simulink model "CATSS_Functional"  (R2025b)
settings: Solver=VariableStepAuto  StartTime=0.0  StopTime=10.0  RelTol=1e-3
settings Model: DataDictionary=CATSS_FunctionalInterfaces.sldd  Creator=sarah  LastModifiedBy=sarah

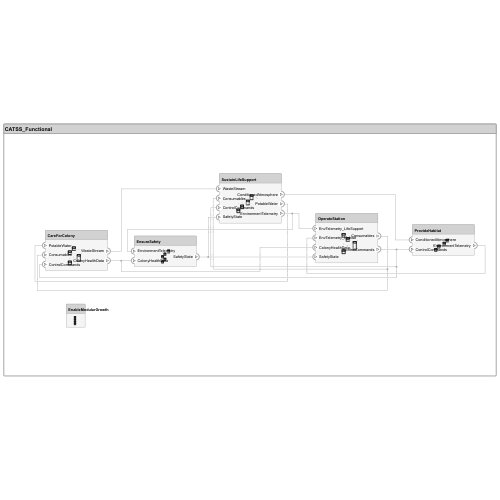
[thumbnail: Simulink's stored preview of the top-level diagram]
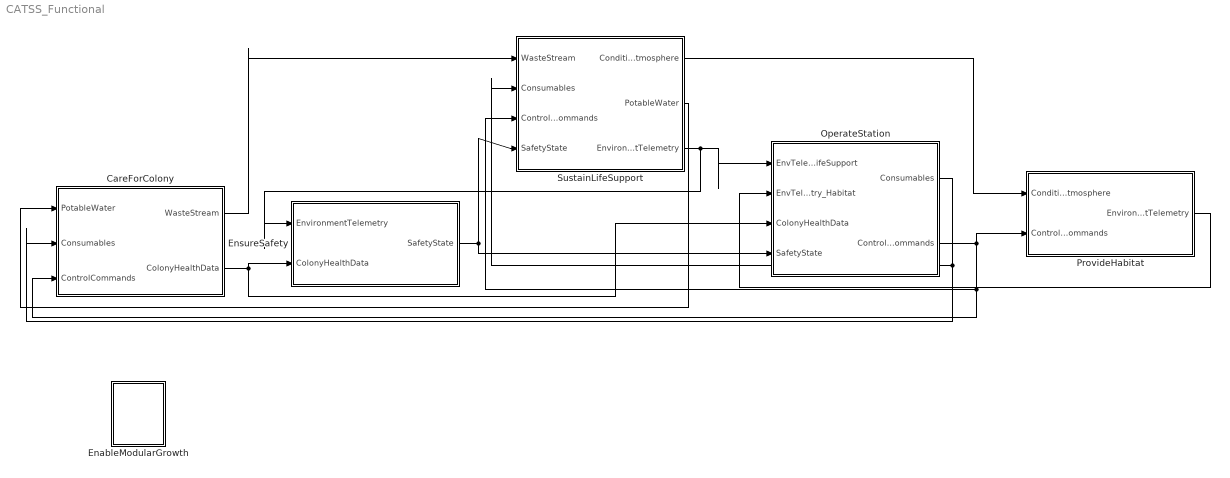
== system CATSS_Functional ==
  CareForColony : Subsystem
      settings: PortSchema="{\"entries\":[{\"content\":{\"headerSize\":26,\"margin\":15,\"minimumSpacing\":25,\"sides\":[{\"content\":{\"connectorIds\":[\"In1\",\"In2\",\"In3\"]},\"type\":\"ConnectorPlacement.EquallySpacedRectSide\",\"uuid\":\"ee9d823c-b058-498d-a1d2-354a2dfab86e\"},{\"content\":{\"connectorIds\":[\"Out1\",\"Out2\"],\"side\":\"RIGHT\"},\"type\":\"ConnectorPlacement.EquallySpacedRectSide\",\"uuid\":\"e3604748-6574-46d6-a392-50dc4429d0e1\"},{\"content\":{\"side\":\"TOP\"},\"type\":\"ConnectorPlacement.EquallySpacedRectSide\",\"uuid\":\"eee796a1-5b1d-4047-be0b-af9e6bf06bf5\"}]},\"type\":\"ConnectorPlacement.EquallySpacedConnector\",\"uuid\":\"95a9b6eb-cbb6-45d0-9b2f-8eab5ca43efc\"}],\"packageUris\":[\"http://schema.mathworks.com/mf0/Connector/R2020b\"],\"version\":\"1.0\"}"
  EnableModularGrowth : Subsystem
      settings: PortSchema="{\"entries\":[{\"content\":{\"headerSize\":26,\"margin\":15,\"minimumSpacing\":25,\"sides\":[{\"content\":{},\"type\":\"ConnectorPlacement.EquallySpacedRectSide\",\"uuid\":\"ee9d823c-b058-498d-a1d2-354a2dfab86e\"},{\"content\":{\"side\":\"RIGHT\"},\"type\":\"ConnectorPlacement.EquallySpacedRectSide\",\"uuid\":\"e3604748-6574-46d6-a392-50dc4429d0e1\"},{\"content\":{\"side\":\"TOP\"},\"type\":\"ConnectorPlacement.EquallySpacedRectSide\",\"uuid\":\"eee796a1-5b1d-4047-be0b-af9e6bf06bf5\"}]},\"type\":\"ConnectorPlacement.EquallySpacedConnector\",\"uuid\":\"95a9b6eb-cbb6-45d0-9b2f-8eab5ca43efc\"}],\"packageUris\":[\"http://schema.mathworks.com/mf0/Connector/R2020b\"],\"version\":\"1.0\"}"
  EnsureSafety : Subsystem
      settings: PortSchema="{\"entries\":[{\"content\":{\"headerSize\":26,\"margin\":15,\"minimumSpacing\":25,\"sides\":[{\"content\":{\"connectorIds\":[\"In1\",\"In2\"]},\"type\":\"ConnectorPlacement.EquallySpacedRectSide\",\"uuid\":\"ee9d823c-b058-498d-a1d2-354a2dfab86e\"},{\"content\":{\"connectorIds\":[\"Out1\"],\"side\":\"RIGHT\"},\"type\":\"ConnectorPlacement.EquallySpacedRectSide\",\"uuid\":\"e3604748-6574-46d6-a392-50dc4429d0e1\"},{\"content\":{\"side\":\"TOP\"},\"type\":\"ConnectorPlacement.EquallySpacedRectSide\",\"uuid\":\"eee796a1-5b1d-4047-be0b-af9e6bf06bf5\"}]},\"type\":\"ConnectorPlacement.EquallySpacedConnector\",\"uuid\":\"95a9b6eb-cbb6-45d0-9b2f-8eab5ca43efc\"}],\"packageUris\":[\"http://schema.mathworks.com/mf0/Connector/R2020b\"],\"version\":\"1.0\"}"
  OperateStation : Subsystem
      settings: PortSchema="{\"entries\":[{\"content\":{\"headerSize\":26,\"margin\":15,\"minimumSpacing\":25,\"sides\":[{\"content\":{\"connectorIds\":[\"In1\",\"In2\",\"In3\",\"In4\"]},\"type\":\"ConnectorPlacement.EquallySpacedRectSide\",\"uuid\":\"ee9d823c-b058-498d-a1d2-354a2dfab86e\"},{\"content\":{\"connectorIds\":[\"Out1\",\"Out2\"],\"side\":\"RIGHT\"},\"type\":\"ConnectorPlacement.EquallySpacedRectSide\",\"uuid\":\"e3604748-6574-46d6-a392-50dc4429d0e1\"},{\"content\":{\"side\":\"TOP\"},\"type\":\"ConnectorPlacement.EquallySpacedRectSide\",\"uuid\":\"eee796a1-5b1d-4047-be0b-af9e6bf06bf5\"}]},\"type\":\"ConnectorPlacement.EquallySpacedConnector\",\"uuid\":\"95a9b6eb-cbb6-45d0-9b2f-8eab5ca43efc\"}],\"packageUris\":[\"http://schema.mathworks.com/mf0/Connector/R2020b\"],\"version\":\"1.0\"}"
  ProvideHabitat : Subsystem
      settings: PortSchema="{\"entries\":[{\"content\":{\"headerSize\":26,\"margin\":15,\"minimumSpacing\":25,\"sides\":[{\"content\":{\"connectorIds\":[\"In1\",\"In2\"]},\"type\":\"ConnectorPlacement.EquallySpacedRectSide\",\"uuid\":\"ee9d823c-b058-498d-a1d2-354a2dfab86e\"},{\"content\":{\"connectorIds\":[\"Out1\"],\"side\":\"RIGHT\"},\"type\":\"ConnectorPlacement.EquallySpacedRectSide\",\"uuid\":\"e3604748-6574-46d6-a392-50dc4429d0e1\"},{\"content\":{\"side\":\"TOP\"},\"type\":\"ConnectorPlacement.EquallySpacedRectSide\",\"uuid\":\"eee796a1-5b1d-4047-be0b-af9e6bf06bf5\"}]},\"type\":\"ConnectorPlacement.EquallySpacedConnector\",\"uuid\":\"95a9b6eb-cbb6-45d0-9b2f-8eab5ca43efc\"}],\"packageUris\":[\"http://schema.mathworks.com/mf0/Connector/R2020b\"],\"version\":\"1.0\"}"
  SustainLifeSupport : Subsystem
      settings: PortSchema="{\"entries\":[{\"content\":{\"headerSize\":26,\"margin\":15,\"minimumSpacing\":25,\"sides\":[{\"content\":{\"connectorIds\":[\"In1\",\"In2\",\"In3\",\"In4\"]},\"type\":\"ConnectorPlacement.EquallySpacedRectSide\",\"uuid\":\"ee9d823c-b058-498d-a1d2-354a2dfab86e\"},{\"content\":{\"connectorIds\":[\"Out1\",\"Out2\",\"Out3\"],\"side\":\"RIGHT\"},\"type\":\"ConnectorPlacement.EquallySpacedRectSide\",\"uuid\":\"e3604748-6574-46d6-a392-50dc4429d0e1\"},{\"content\":{\"side\":\"TOP\"},\"type\":\"ConnectorPlacement.EquallySpacedRectSide\",\"uuid\":\"eee796a1-5b1d-4047-be0b-af9e6bf06bf5\"}]},\"type\":\"ConnectorPlacement.EquallySpacedConnector\",\"uuid\":\"95a9b6eb-cbb6-45d0-9b2f-8eab5ca43efc\"}],\"packageUris\":[\"http://schema.mathworks.com/mf0/Connector/R2020b\"],\"version\":\"1.0\"}"
  wires:
  EnsureSafety/1(SafetyState) -> SustainLifeSupport/4(SafetyState), OperateStation/4(SafetyState)
  OperateStation/2(ControlCommands) -> CareForColony/3(ControlCommands), SustainLifeSupport/3(ControlCommands), ProvideHabitat/2(ControlCommands)
  OperateStation/1(Consumables) -> CareForColony/2(Consumables), SustainLifeSupport/2(Consumables)
  ProvideHabitat/1(EnvironmentTelemetry) -> OperateStation/2(EnvTelemetry_Habitat)
  CareForColony/2(ColonyHealthData) -> EnsureSafety/2(ColonyHealthData), OperateStation/3(ColonyHealthData)
  CareForColony/1(WasteStream) -> SustainLifeSupport/1(WasteStream)
  SustainLifeSupport/3(EnvironmentTelemetry) -> EnsureSafety/1(EnvironmentTelemetry), OperateStation/1(EnvTelemetry_LifeSupport)
  SustainLifeSupport/2(PotableWater) -> CareForColony/1(PotableWater)
  SustainLifeSupport/1(ConditionedAtmosphere) -> ProvideHabitat/1(ConditionedAtmosphere)

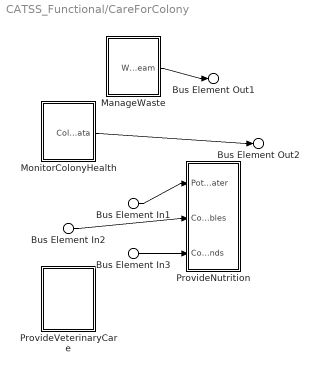
== system CATSS_Functional/CareForColony ==
  Bus Element In1 : Inport  PortName=PotableWater
  Bus Element In2 : Inport  Port=2  PortName=Consumables
  Bus Element In3 : Inport  Port=3  PortName=ControlCommands
  ManageWaste : Subsystem
      settings: PortSchema="{\"entries\":[{\"content\":{\"headerSize\":26,\"margin\":15,\"minimumSpacing\":25,\"sides\":[{\"content\":{},\"type\":\"ConnectorPlacement.EquallySpacedRectSide\",\"uuid\":\"ee9d823c-b058-498d-a1d2-354a2dfab86e\"},{\"content\":{\"connectorIds\":[\"Out1\"],\"side\":\"RIGHT\"},\"type\":\"ConnectorPlacement.EquallySpacedRectSide\",\"uuid\":\"e3604748-6574-46d6-a392-50dc4429d0e1\"},{\"content\":{\"side\":\"TOP\"},\"type\":\"ConnectorPlacement.EquallySpacedRectSide\",\"uuid\":\"eee796a1-5b1d-4047-be0b-af9e6bf06bf5\"}]},\"type\":\"ConnectorPlacement.EquallySpacedConnector\",\"uuid\":\"95a9b6eb-cbb6-45d0-9b2f-8eab5ca43efc\"}],\"packageUris\":[\"http://schema.mathworks.com/mf0/Connector/R2020b\"],\"version\":\"1.0\"}"
  MonitorColonyHealth : Subsystem
      settings: PortSchema="{\"entries\":[{\"content\":{\"headerSize\":26,\"margin\":15,\"minimumSpacing\":25,\"sides\":[{\"content\":{},\"type\":\"ConnectorPlacement.EquallySpacedRectSide\",\"uuid\":\"ee9d823c-b058-498d-a1d2-354a2dfab86e\"},{\"content\":{\"connectorIds\":[\"Out1\"],\"side\":\"RIGHT\"},\"type\":\"ConnectorPlacement.EquallySpacedRectSide\",\"uuid\":\"e3604748-6574-46d6-a392-50dc4429d0e1\"},{\"content\":{\"side\":\"TOP\"},\"type\":\"ConnectorPlacement.EquallySpacedRectSide\",\"uuid\":\"eee796a1-5b1d-4047-be0b-af9e6bf06bf5\"}]},\"type\":\"ConnectorPlacement.EquallySpacedConnector\",\"uuid\":\"95a9b6eb-cbb6-45d0-9b2f-8eab5ca43efc\"}],\"packageUris\":[\"http://schema.mathworks.com/mf0/Connector/R2020b\"],\"version\":\"1.0\"}"
  ProvideNutrition : Subsystem
      settings: PortSchema="{\"entries\":[{\"content\":{\"headerSize\":26,\"margin\":15,\"minimumSpacing\":25,\"sides\":[{\"content\":{\"connectorIds\":[\"In1\",\"In2\",\"In3\"]},\"type\":\"ConnectorPlacement.EquallySpacedRectSide\",\"uuid\":\"ee9d823c-b058-498d-a1d2-354a2dfab86e\"},{\"content\":{\"side\":\"RIGHT\"},\"type\":\"ConnectorPlacement.EquallySpacedRectSide\",\"uuid\":\"e3604748-6574-46d6-a392-50dc4429d0e1\"},{\"content\":{\"side\":\"TOP\"},\"type\":\"ConnectorPlacement.EquallySpacedRectSide\",\"uuid\":\"eee796a1-5b1d-4047-be0b-af9e6bf06bf5\"}]},\"type\":\"ConnectorPlacement.EquallySpacedConnector\",\"uuid\":\"95a9b6eb-cbb6-45d0-9b2f-8eab5ca43efc\"}],\"packageUris\":[\"http://schema.mathworks.com/mf0/Connector/R2020b\"],\"version\":\"1.0\"}"
  ProvideVeterinaryCare : Subsystem
      settings: PortSchema="{\"entries\":[{\"content\":{\"headerSize\":26,\"margin\":15,\"minimumSpacing\":25,\"sides\":[{\"content\":{},\"type\":\"ConnectorPlacement.EquallySpacedRectSide\",\"uuid\":\"ee9d823c-b058-498d-a1d2-354a2dfab86e\"},{\"content\":{\"side\":\"RIGHT\"},\"type\":\"ConnectorPlacement.EquallySpacedRectSide\",\"uuid\":\"e3604748-6574-46d6-a392-50dc4429d0e1\"},{\"content\":{\"side\":\"TOP\"},\"type\":\"ConnectorPlacement.EquallySpacedRectSide\",\"uuid\":\"eee796a1-5b1d-4047-be0b-af9e6bf06bf5\"}]},\"type\":\"ConnectorPlacement.EquallySpacedConnector\",\"uuid\":\"95a9b6eb-cbb6-45d0-9b2f-8eab5ca43efc\"}],\"packageUris\":[\"http://schema.mathworks.com/mf0/Connector/R2020b\"],\"version\":\"1.0\"}"
  Bus Element Out1 : Outport  PortName=WasteStream
  Bus Element Out2 : Outport  Port=2  PortName=ColonyHealthData
  wires:
  MonitorColonyHealth/1(ColonyHealthData) -> Bus Element Out2/1
  ManageWaste/1(WasteStream) -> Bus Element Out1/1
  Bus Element In3/1 -> ProvideNutrition/3(ControlCommands)
  Bus Element In2/1 -> ProvideNutrition/2(Consumables)
  Bus Element In1/1 -> ProvideNutrition/1(PotableWater)

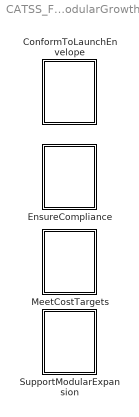
== system CATSS_Functional/EnableModularGrowth ==
  ConformToLaunchEnvelope : Subsystem
      settings: PortSchema="{\"entries\":[{\"content\":{\"headerSize\":26,\"margin\":15,\"minimumSpacing\":25,\"sides\":[{\"content\":{},\"type\":\"ConnectorPlacement.EquallySpacedRectSide\",\"uuid\":\"ee9d823c-b058-498d-a1d2-354a2dfab86e\"},{\"content\":{\"side\":\"RIGHT\"},\"type\":\"ConnectorPlacement.EquallySpacedRectSide\",\"uuid\":\"e3604748-6574-46d6-a392-50dc4429d0e1\"},{\"content\":{\"side\":\"TOP\"},\"type\":\"ConnectorPlacement.EquallySpacedRectSide\",\"uuid\":\"eee796a1-5b1d-4047-be0b-af9e6bf06bf5\"}]},\"type\":\"ConnectorPlacement.EquallySpacedConnector\",\"uuid\":\"95a9b6eb-cbb6-45d0-9b2f-8eab5ca43efc\"}],\"packageUris\":[\"http://schema.mathworks.com/mf0/Connector/R2020b\"],\"version\":\"1.0\"}"
  EnsureCompliance : Subsystem
      settings: PortSchema="{\"entries\":[{\"content\":{\"headerSize\":26,\"margin\":15,\"minimumSpacing\":25,\"sides\":[{\"content\":{},\"type\":\"ConnectorPlacement.EquallySpacedRectSide\",\"uuid\":\"ee9d823c-b058-498d-a1d2-354a2dfab86e\"},{\"content\":{\"side\":\"RIGHT\"},\"type\":\"ConnectorPlacement.EquallySpacedRectSide\",\"uuid\":\"e3604748-6574-46d6-a392-50dc4429d0e1\"},{\"content\":{\"side\":\"TOP\"},\"type\":\"ConnectorPlacement.EquallySpacedRectSide\",\"uuid\":\"eee796a1-5b1d-4047-be0b-af9e6bf06bf5\"}]},\"type\":\"ConnectorPlacement.EquallySpacedConnector\",\"uuid\":\"95a9b6eb-cbb6-45d0-9b2f-8eab5ca43efc\"}],\"packageUris\":[\"http://schema.mathworks.com/mf0/Connector/R2020b\"],\"version\":\"1.0\"}"
  MeetCostTargets : Subsystem
      settings: PortSchema="{\"entries\":[{\"content\":{\"headerSize\":26,\"margin\":15,\"minimumSpacing\":25,\"sides\":[{\"content\":{},\"type\":\"ConnectorPlacement.EquallySpacedRectSide\",\"uuid\":\"ee9d823c-b058-498d-a1d2-354a2dfab86e\"},{\"content\":{\"side\":\"RIGHT\"},\"type\":\"ConnectorPlacement.EquallySpacedRectSide\",\"uuid\":\"e3604748-6574-46d6-a392-50dc4429d0e1\"},{\"content\":{\"side\":\"TOP\"},\"type\":\"ConnectorPlacement.EquallySpacedRectSide\",\"uuid\":\"eee796a1-5b1d-4047-be0b-af9e6bf06bf5\"}]},\"type\":\"ConnectorPlacement.EquallySpacedConnector\",\"uuid\":\"95a9b6eb-cbb6-45d0-9b2f-8eab5ca43efc\"}],\"packageUris\":[\"http://schema.mathworks.com/mf0/Connector/R2020b\"],\"version\":\"1.0\"}"
  SupportModularExpansion : Subsystem
      settings: PortSchema="{\"entries\":[{\"content\":{\"headerSize\":26,\"margin\":15,\"minimumSpacing\":25,\"sides\":[{\"content\":{},\"type\":\"ConnectorPlacement.EquallySpacedRectSide\",\"uuid\":\"ee9d823c-b058-498d-a1d2-354a2dfab86e\"},{\"content\":{\"side\":\"RIGHT\"},\"type\":\"ConnectorPlacement.EquallySpacedRectSide\",\"uuid\":\"e3604748-6574-46d6-a392-50dc4429d0e1\"},{\"content\":{\"side\":\"TOP\"},\"type\":\"ConnectorPlacement.EquallySpacedRectSide\",\"uuid\":\"eee796a1-5b1d-4047-be0b-af9e6bf06bf5\"}]},\"type\":\"ConnectorPlacement.EquallySpacedConnector\",\"uuid\":\"95a9b6eb-cbb6-45d0-9b2f-8eab5ca43efc\"}],\"packageUris\":[\"http://schema.mathworks.com/mf0/Connector/R2020b\"],\"version\":\"1.0\"}"

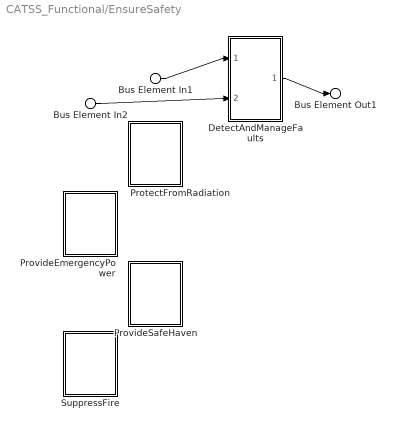
== system CATSS_Functional/EnsureSafety ==
  Bus Element In1 : Inport  PortName=EnvironmentTelemetry
  Bus Element In2 : Inport  Port=2  PortName=ColonyHealthData
  DetectAndManageFaults : Subsystem
      settings: PortSchema="{\"entries\":[{\"content\":{\"headerSize\":26,\"margin\":15,\"minimumSpacing\":25,\"sides\":[{\"content\":{\"connectorIds\":[\"In1\",\"In2\"]},\"type\":\"ConnectorPlacement.EquallySpacedRectSide\",\"uuid\":\"ee9d823c-b058-498d-a1d2-354a2dfab86e\"},{\"content\":{\"connectorIds\":[\"Out1\"],\"side\":\"RIGHT\"},\"type\":\"ConnectorPlacement.EquallySpacedRectSide\",\"uuid\":\"e3604748-6574-46d6-a392-50dc4429d0e1\"},{\"content\":{\"side\":\"TOP\"},\"type\":\"ConnectorPlacement.EquallySpacedRectSide\",\"uuid\":\"eee796a1-5b1d-4047-be0b-af9e6bf06bf5\"}]},\"type\":\"ConnectorPlacement.EquallySpacedConnector\",\"uuid\":\"95a9b6eb-cbb6-45d0-9b2f-8eab5ca43efc\"}],\"packageUris\":[\"http://schema.mathworks.com/mf0/Connector/R2020b\"],\"version\":\"1.0\"}"
  ProtectFromRadiation : Subsystem
      settings: PortSchema="{\"entries\":[{\"content\":{\"headerSize\":26,\"margin\":15,\"minimumSpacing\":25,\"sides\":[{\"content\":{},\"type\":\"ConnectorPlacement.EquallySpacedRectSide\",\"uuid\":\"ee9d823c-b058-498d-a1d2-354a2dfab86e\"},{\"content\":{\"side\":\"RIGHT\"},\"type\":\"ConnectorPlacement.EquallySpacedRectSide\",\"uuid\":\"e3604748-6574-46d6-a392-50dc4429d0e1\"},{\"content\":{\"side\":\"TOP\"},\"type\":\"ConnectorPlacement.EquallySpacedRectSide\",\"uuid\":\"eee796a1-5b1d-4047-be0b-af9e6bf06bf5\"}]},\"type\":\"ConnectorPlacement.EquallySpacedConnector\",\"uuid\":\"95a9b6eb-cbb6-45d0-9b2f-8eab5ca43efc\"}],\"packageUris\":[\"http://schema.mathworks.com/mf0/Connector/R2020b\"],\"version\":\"1.0\"}"
  ProvideEmergencyPower : Subsystem
      settings: PortSchema="{\"entries\":[{\"content\":{\"headerSize\":26,\"margin\":15,\"minimumSpacing\":25,\"sides\":[{\"content\":{},\"type\":\"ConnectorPlacement.EquallySpacedRectSide\",\"uuid\":\"ee9d823c-b058-498d-a1d2-354a2dfab86e\"},{\"content\":{\"side\":\"RIGHT\"},\"type\":\"ConnectorPlacement.EquallySpacedRectSide\",\"uuid\":\"e3604748-6574-46d6-a392-50dc4429d0e1\"},{\"content\":{\"side\":\"TOP\"},\"type\":\"ConnectorPlacement.EquallySpacedRectSide\",\"uuid\":\"eee796a1-5b1d-4047-be0b-af9e6bf06bf5\"}]},\"type\":\"ConnectorPlacement.EquallySpacedConnector\",\"uuid\":\"95a9b6eb-cbb6-45d0-9b2f-8eab5ca43efc\"}],\"packageUris\":[\"http://schema.mathworks.com/mf0/Connector/R2020b\"],\"version\":\"1.0\"}"
  ProvideSafeHaven : Subsystem
      settings: PortSchema="{\"entries\":[{\"content\":{\"headerSize\":26,\"margin\":15,\"minimumSpacing\":25,\"sides\":[{\"content\":{},\"type\":\"ConnectorPlacement.EquallySpacedRectSide\",\"uuid\":\"ee9d823c-b058-498d-a1d2-354a2dfab86e\"},{\"content\":{\"side\":\"RIGHT\"},\"type\":\"ConnectorPlacement.EquallySpacedRectSide\",\"uuid\":\"e3604748-6574-46d6-a392-50dc4429d0e1\"},{\"content\":{\"side\":\"TOP\"},\"type\":\"ConnectorPlacement.EquallySpacedRectSide\",\"uuid\":\"eee796a1-5b1d-4047-be0b-af9e6bf06bf5\"}]},\"type\":\"ConnectorPlacement.EquallySpacedConnector\",\"uuid\":\"95a9b6eb-cbb6-45d0-9b2f-8eab5ca43efc\"}],\"packageUris\":[\"http://schema.mathworks.com/mf0/Connector/R2020b\"],\"version\":\"1.0\"}"
  SuppressFire : Subsystem
      settings: PortSchema="{\"entries\":[{\"content\":{\"headerSize\":26,\"margin\":15,\"minimumSpacing\":25,\"sides\":[{\"content\":{},\"type\":\"ConnectorPlacement.EquallySpacedRectSide\",\"uuid\":\"ee9d823c-b058-498d-a1d2-354a2dfab86e\"},{\"content\":{\"side\":\"RIGHT\"},\"type\":\"ConnectorPlacement.EquallySpacedRectSide\",\"uuid\":\"e3604748-6574-46d6-a392-50dc4429d0e1\"},{\"content\":{\"side\":\"TOP\"},\"type\":\"ConnectorPlacement.EquallySpacedRectSide\",\"uuid\":\"eee796a1-5b1d-4047-be0b-af9e6bf06bf5\"}]},\"type\":\"ConnectorPlacement.EquallySpacedConnector\",\"uuid\":\"95a9b6eb-cbb6-45d0-9b2f-8eab5ca43efc\"}],\"packageUris\":[\"http://schema.mathworks.com/mf0/Connector/R2020b\"],\"version\":\"1.0\"}"
  Bus Element Out1 : Outport  PortName=SafetyState
  wires:
  DetectAndManageFaults/1(SafetyState) -> Bus Element Out1/1
  Bus Element In2/1 -> DetectAndManageFaults/2(ColonyHealthData)
  Bus Element In1/1 -> DetectAndManageFaults/1(EnvironmentTelemetry)

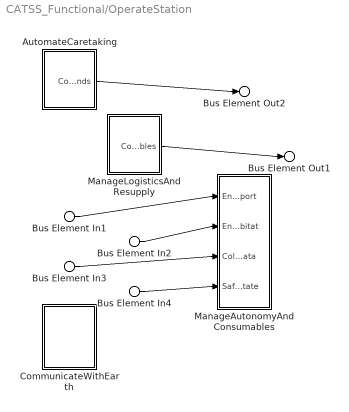
== system CATSS_Functional/OperateStation ==
  Bus Element In1 : Inport  PortName=EnvTelemetry_LifeSupport
  Bus Element In2 : Inport  Port=2  PortName=EnvTelemetry_Habitat
  Bus Element In3 : Inport  Port=3  PortName=ColonyHealthData
  Bus Element In4 : Inport  Port=4  PortName=SafetyState
  AutomateCaretaking : Subsystem
      settings: PortSchema="{\"entries\":[{\"content\":{\"headerSize\":26,\"margin\":15,\"minimumSpacing\":25,\"sides\":[{\"content\":{},\"type\":\"ConnectorPlacement.EquallySpacedRectSide\",\"uuid\":\"ee9d823c-b058-498d-a1d2-354a2dfab86e\"},{\"content\":{\"connectorIds\":[\"Out1\"],\"side\":\"RIGHT\"},\"type\":\"ConnectorPlacement.EquallySpacedRectSide\",\"uuid\":\"e3604748-6574-46d6-a392-50dc4429d0e1\"},{\"content\":{\"side\":\"TOP\"},\"type\":\"ConnectorPlacement.EquallySpacedRectSide\",\"uuid\":\"eee796a1-5b1d-4047-be0b-af9e6bf06bf5\"}]},\"type\":\"ConnectorPlacement.EquallySpacedConnector\",\"uuid\":\"95a9b6eb-cbb6-45d0-9b2f-8eab5ca43efc\"}],\"packageUris\":[\"http://schema.mathworks.com/mf0/Connector/R2020b\"],\"version\":\"1.0\"}"
  CommunicateWithEarth : Subsystem
      settings: PortSchema="{\"entries\":[{\"content\":{\"headerSize\":26,\"margin\":15,\"minimumSpacing\":25,\"sides\":[{\"content\":{},\"type\":\"ConnectorPlacement.EquallySpacedRectSide\",\"uuid\":\"ee9d823c-b058-498d-a1d2-354a2dfab86e\"},{\"content\":{\"side\":\"RIGHT\"},\"type\":\"ConnectorPlacement.EquallySpacedRectSide\",\"uuid\":\"e3604748-6574-46d6-a392-50dc4429d0e1\"},{\"content\":{\"side\":\"TOP\"},\"type\":\"ConnectorPlacement.EquallySpacedRectSide\",\"uuid\":\"eee796a1-5b1d-4047-be0b-af9e6bf06bf5\"}]},\"type\":\"ConnectorPlacement.EquallySpacedConnector\",\"uuid\":\"95a9b6eb-cbb6-45d0-9b2f-8eab5ca43efc\"}],\"packageUris\":[\"http://schema.mathworks.com/mf0/Connector/R2020b\"],\"version\":\"1.0\"}"
  ManageAutonomyAndConsumables : Subsystem
      settings: PortSchema="{\"entries\":[{\"content\":{\"headerSize\":26,\"margin\":15,\"minimumSpacing\":25,\"sides\":[{\"content\":{\"connectorIds\":[\"In1\",\"In2\",\"In3\",\"In4\"]},\"type\":\"ConnectorPlacement.EquallySpacedRectSide\",\"uuid\":\"ee9d823c-b058-498d-a1d2-354a2dfab86e\"},{\"content\":{\"side\":\"RIGHT\"},\"type\":\"ConnectorPlacement.EquallySpacedRectSide\",\"uuid\":\"e3604748-6574-46d6-a392-50dc4429d0e1\"},{\"content\":{\"side\":\"TOP\"},\"type\":\"ConnectorPlacement.EquallySpacedRectSide\",\"uuid\":\"eee796a1-5b1d-4047-be0b-af9e6bf06bf5\"}]},\"type\":\"ConnectorPlacement.EquallySpacedConnector\",\"uuid\":\"95a9b6eb-cbb6-45d0-9b2f-8eab5ca43efc\"}],\"packageUris\":[\"http://schema.mathworks.com/mf0/Connector/R2020b\"],\"version\":\"1.0\"}"
  ManageLogisticsAndResupply : Subsystem
      settings: PortSchema="{\"entries\":[{\"content\":{\"headerSize\":26,\"margin\":15,\"minimumSpacing\":25,\"sides\":[{\"content\":{},\"type\":\"ConnectorPlacement.EquallySpacedRectSide\",\"uuid\":\"ee9d823c-b058-498d-a1d2-354a2dfab86e\"},{\"content\":{\"connectorIds\":[\"Out1\"],\"side\":\"RIGHT\"},\"type\":\"ConnectorPlacement.EquallySpacedRectSide\",\"uuid\":\"e3604748-6574-46d6-a392-50dc4429d0e1\"},{\"content\":{\"side\":\"TOP\"},\"type\":\"ConnectorPlacement.EquallySpacedRectSide\",\"uuid\":\"eee796a1-5b1d-4047-be0b-af9e6bf06bf5\"}]},\"type\":\"ConnectorPlacement.EquallySpacedConnector\",\"uuid\":\"95a9b6eb-cbb6-45d0-9b2f-8eab5ca43efc\"}],\"packageUris\":[\"http://schema.mathworks.com/mf0/Connector/R2020b\"],\"version\":\"1.0\"}"
  Bus Element Out1 : Outport  PortName=Consumables
  Bus Element Out2 : Outport  Port=2  PortName=ControlCommands
  wires:
  AutomateCaretaking/1(ControlCommands) -> Bus Element Out2/1
  ManageLogisticsAndResupply/1(Consumables) -> Bus Element Out1/1
  Bus Element In4/1 -> ManageAutonomyAndConsumables/4(SafetyState)
  Bus Element In3/1 -> ManageAutonomyAndConsumables/3(ColonyHealthData)
  Bus Element In2/1 -> ManageAutonomyAndConsumables/2(EnvTelemetry_Habitat)
  Bus Element In1/1 -> ManageAutonomyAndConsumables/1(EnvTelemetry_LifeSupport)

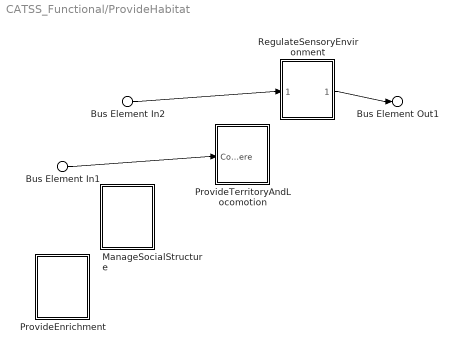
== system CATSS_Functional/ProvideHabitat ==
  Bus Element In1 : Inport  PortName=ConditionedAtmosphere
  Bus Element In2 : Inport  Port=2  PortName=ControlCommands
  ManageSocialStructure : Subsystem
      settings: PortSchema="{\"entries\":[{\"content\":{\"headerSize\":26,\"margin\":15,\"minimumSpacing\":25,\"sides\":[{\"content\":{},\"type\":\"ConnectorPlacement.EquallySpacedRectSide\",\"uuid\":\"ee9d823c-b058-498d-a1d2-354a2dfab86e\"},{\"content\":{\"side\":\"RIGHT\"},\"type\":\"ConnectorPlacement.EquallySpacedRectSide\",\"uuid\":\"e3604748-6574-46d6-a392-50dc4429d0e1\"},{\"content\":{\"side\":\"TOP\"},\"type\":\"ConnectorPlacement.EquallySpacedRectSide\",\"uuid\":\"eee796a1-5b1d-4047-be0b-af9e6bf06bf5\"}]},\"type\":\"ConnectorPlacement.EquallySpacedConnector\",\"uuid\":\"95a9b6eb-cbb6-45d0-9b2f-8eab5ca43efc\"}],\"packageUris\":[\"http://schema.mathworks.com/mf0/Connector/R2020b\"],\"version\":\"1.0\"}"
  ProvideEnrichment : Subsystem
      settings: PortSchema="{\"entries\":[{\"content\":{\"headerSize\":26,\"margin\":15,\"minimumSpacing\":25,\"sides\":[{\"content\":{},\"type\":\"ConnectorPlacement.EquallySpacedRectSide\",\"uuid\":\"ee9d823c-b058-498d-a1d2-354a2dfab86e\"},{\"content\":{\"side\":\"RIGHT\"},\"type\":\"ConnectorPlacement.EquallySpacedRectSide\",\"uuid\":\"e3604748-6574-46d6-a392-50dc4429d0e1\"},{\"content\":{\"side\":\"TOP\"},\"type\":\"ConnectorPlacement.EquallySpacedRectSide\",\"uuid\":\"eee796a1-5b1d-4047-be0b-af9e6bf06bf5\"}]},\"type\":\"ConnectorPlacement.EquallySpacedConnector\",\"uuid\":\"95a9b6eb-cbb6-45d0-9b2f-8eab5ca43efc\"}],\"packageUris\":[\"http://schema.mathworks.com/mf0/Connector/R2020b\"],\"version\":\"1.0\"}"
  ProvideTerritoryAndLocomotion : Subsystem
      settings: PortSchema="{\"entries\":[{\"content\":{\"headerSize\":26,\"margin\":15,\"minimumSpacing\":25,\"sides\":[{\"content\":{\"connectorIds\":[\"In1\"]},\"type\":\"ConnectorPlacement.EquallySpacedRectSide\",\"uuid\":\"ee9d823c-b058-498d-a1d2-354a2dfab86e\"},{\"content\":{\"side\":\"RIGHT\"},\"type\":\"ConnectorPlacement.EquallySpacedRectSide\",\"uuid\":\"e3604748-6574-46d6-a392-50dc4429d0e1\"},{\"content\":{\"side\":\"TOP\"},\"type\":\"ConnectorPlacement.EquallySpacedRectSide\",\"uuid\":\"eee796a1-5b1d-4047-be0b-af9e6bf06bf5\"}]},\"type\":\"ConnectorPlacement.EquallySpacedConnector\",\"uuid\":\"95a9b6eb-cbb6-45d0-9b2f-8eab5ca43efc\"}],\"packageUris\":[\"http://schema.mathworks.com/mf0/Connector/R2020b\"],\"version\":\"1.0\"}"
  RegulateSensoryEnvironment : Subsystem
      settings: PortSchema="{\"entries\":[{\"content\":{\"headerSize\":26,\"margin\":15,\"minimumSpacing\":25,\"sides\":[{\"content\":{\"connectorIds\":[\"In1\"]},\"type\":\"ConnectorPlacement.EquallySpacedRectSide\",\"uuid\":\"ee9d823c-b058-498d-a1d2-354a2dfab86e\"},{\"content\":{\"connectorIds\":[\"Out1\"],\"side\":\"RIGHT\"},\"type\":\"ConnectorPlacement.EquallySpacedRectSide\",\"uuid\":\"e3604748-6574-46d6-a392-50dc4429d0e1\"},{\"content\":{\"side\":\"TOP\"},\"type\":\"ConnectorPlacement.EquallySpacedRectSide\",\"uuid\":\"eee796a1-5b1d-4047-be0b-af9e6bf06bf5\"}]},\"type\":\"ConnectorPlacement.EquallySpacedConnector\",\"uuid\":\"95a9b6eb-cbb6-45d0-9b2f-8eab5ca43efc\"}],\"packageUris\":[\"http://schema.mathworks.com/mf0/Connector/R2020b\"],\"version\":\"1.0\"}"
  Bus Element Out1 : Outport  PortName=EnvironmentTelemetry
  wires:
  RegulateSensoryEnvironment/1(EnvironmentTelemetry) -> Bus Element Out1/1
  Bus Element In2/1 -> RegulateSensoryEnvironment/1(ControlCommands)
  Bus Element In1/1 -> ProvideTerritoryAndLocomotion/1(ConditionedAtmosphere)

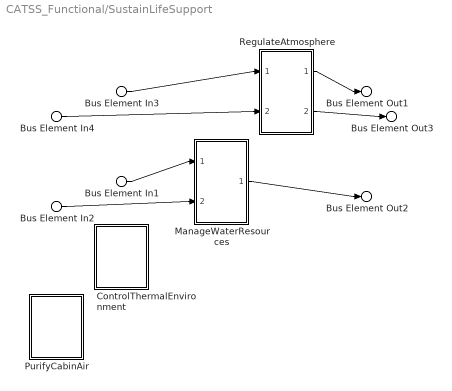
== system CATSS_Functional/SustainLifeSupport ==
  Bus Element In1 : Inport  PortName=WasteStream
  Bus Element In2 : Inport  Port=2  PortName=Consumables
  Bus Element In3 : Inport  Port=3  PortName=ControlCommands
  Bus Element In4 : Inport  Port=4  PortName=SafetyState
  ControlThermalEnvironment : Subsystem
      settings: PortSchema="{\"entries\":[{\"content\":{\"headerSize\":26,\"margin\":15,\"minimumSpacing\":25,\"sides\":[{\"content\":{},\"type\":\"ConnectorPlacement.EquallySpacedRectSide\",\"uuid\":\"ee9d823c-b058-498d-a1d2-354a2dfab86e\"},{\"content\":{\"side\":\"RIGHT\"},\"type\":\"ConnectorPlacement.EquallySpacedRectSide\",\"uuid\":\"e3604748-6574-46d6-a392-50dc4429d0e1\"},{\"content\":{\"side\":\"TOP\"},\"type\":\"ConnectorPlacement.EquallySpacedRectSide\",\"uuid\":\"eee796a1-5b1d-4047-be0b-af9e6bf06bf5\"}]},\"type\":\"ConnectorPlacement.EquallySpacedConnector\",\"uuid\":\"95a9b6eb-cbb6-45d0-9b2f-8eab5ca43efc\"}],\"packageUris\":[\"http://schema.mathworks.com/mf0/Connector/R2020b\"],\"version\":\"1.0\"}"
  ManageWaterResources : Subsystem
      settings: PortSchema="{\"entries\":[{\"content\":{\"headerSize\":26,\"margin\":15,\"minimumSpacing\":25,\"sides\":[{\"content\":{\"connectorIds\":[\"In1\",\"In2\"]},\"type\":\"ConnectorPlacement.EquallySpacedRectSide\",\"uuid\":\"ee9d823c-b058-498d-a1d2-354a2dfab86e\"},{\"content\":{\"connectorIds\":[\"Out1\"],\"side\":\"RIGHT\"},\"type\":\"ConnectorPlacement.EquallySpacedRectSide\",\"uuid\":\"e3604748-6574-46d6-a392-50dc4429d0e1\"},{\"content\":{\"side\":\"TOP\"},\"type\":\"ConnectorPlacement.EquallySpacedRectSide\",\"uuid\":\"eee796a1-5b1d-4047-be0b-af9e6bf06bf5\"}]},\"type\":\"ConnectorPlacement.EquallySpacedConnector\",\"uuid\":\"95a9b6eb-cbb6-45d0-9b2f-8eab5ca43efc\"}],\"packageUris\":[\"http://schema.mathworks.com/mf0/Connector/R2020b\"],\"version\":\"1.0\"}"
  PurifyCabinAir : Subsystem
      settings: PortSchema="{\"entries\":[{\"content\":{\"headerSize\":26,\"margin\":15,\"minimumSpacing\":25,\"sides\":[{\"content\":{},\"type\":\"ConnectorPlacement.EquallySpacedRectSide\",\"uuid\":\"ee9d823c-b058-498d-a1d2-354a2dfab86e\"},{\"content\":{\"side\":\"RIGHT\"},\"type\":\"ConnectorPlacement.EquallySpacedRectSide\",\"uuid\":\"e3604748-6574-46d6-a392-50dc4429d0e1\"},{\"content\":{\"side\":\"TOP\"},\"type\":\"ConnectorPlacement.EquallySpacedRectSide\",\"uuid\":\"eee796a1-5b1d-4047-be0b-af9e6bf06bf5\"}]},\"type\":\"ConnectorPlacement.EquallySpacedConnector\",\"uuid\":\"95a9b6eb-cbb6-45d0-9b2f-8eab5ca43efc\"}],\"packageUris\":[\"http://schema.mathworks.com/mf0/Connector/R2020b\"],\"version\":\"1.0\"}"
  RegulateAtmosphere : Subsystem
      settings: PortSchema="{\"entries\":[{\"content\":{\"headerSize\":26,\"margin\":15,\"minimumSpacing\":25,\"sides\":[{\"content\":{\"connectorIds\":[\"In1\",\"In2\"]},\"type\":\"ConnectorPlacement.EquallySpacedRectSide\",\"uuid\":\"ee9d823c-b058-498d-a1d2-354a2dfab86e\"},{\"content\":{\"connectorIds\":[\"Out1\",\"Out2\"],\"side\":\"RIGHT\"},\"type\":\"ConnectorPlacement.EquallySpacedRectSide\",\"uuid\":\"e3604748-6574-46d6-a392-50dc4429d0e1\"},{\"content\":{\"side\":\"TOP\"},\"type\":\"ConnectorPlacement.EquallySpacedRectSide\",\"uuid\":\"eee796a1-5b1d-4047-be0b-af9e6bf06bf5\"}]},\"type\":\"ConnectorPlacement.EquallySpacedConnector\",\"uuid\":\"95a9b6eb-cbb6-45d0-9b2f-8eab5ca43efc\"}],\"packageUris\":[\"http://schema.mathworks.com/mf0/Connector/R2020b\"],\"version\":\"1.0\"}"
  Bus Element Out1 : Outport  PortName=ConditionedAtmosphere
  Bus Element Out2 : Outport  Port=2  PortName=PotableWater
  Bus Element Out3 : Outport  Port=3  PortName=EnvironmentTelemetry
  wires:
  Bus Element In2/1 -> ManageWaterResources/2(Consumables)
  Bus Element In1/1 -> ManageWaterResources/1(WasteStream)
  ManageWaterResources/1(PotableWater) -> Bus Element Out2/1
  RegulateAtmosphere/2(EnvironmentTelemetry) -> Bus Element Out3/1
  Bus Element In4/1 -> RegulateAtmosphere/2(SafetyState)
  Bus Element In3/1 -> RegulateAtmosphere/1(ControlCommands)
  RegulateAtmosphere/1(ConditionedAtmosphere) -> Bus Element Out1/1

== system CATSS_Functional/CareForColony/ManageWaste ==
  Bus Element Out1 : Outport  PortName=WasteStream

== system CATSS_Functional/CareForColony/MonitorColonyHealth ==
  Bus Element Out1 : Outport  PortName=ColonyHealthData

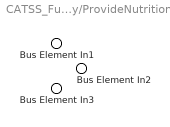
== system CATSS_Functional/CareForColony/ProvideNutrition ==
  Bus Element In1 : Inport  PortName=PotableWater
  Bus Element In2 : Inport  Port=2  PortName=Consumables
  Bus Element In3 : Inport  Port=3  PortName=ControlCommands

== system CATSS_Functional/CareForColony/ProvideVeterinaryCare ==

== system CATSS_Functional/EnableModularGrowth/ConformToLaunchEnvelope ==

== system CATSS_Functional/EnableModularGrowth/EnsureCompliance ==

== system CATSS_Functional/EnableModularGrowth/MeetCostTargets ==

== system CATSS_Functional/EnableModularGrowth/SupportModularExpansion ==

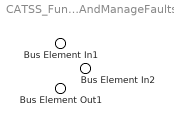
== system CATSS_Functional/EnsureSafety/DetectAndManageFaults ==
  Bus Element In1 : Inport  PortName=EnvironmentTelemetry
  Bus Element In2 : Inport  Port=2  PortName=ColonyHealthData
  Bus Element Out1 : Outport  PortName=SafetyState

== system CATSS_Functional/EnsureSafety/ProtectFromRadiation ==

== system CATSS_Functional/EnsureSafety/ProvideEmergencyPower ==

== system CATSS_Functional/EnsureSafety/ProvideSafeHaven ==

== system CATSS_Functional/EnsureSafety/SuppressFire ==

== system CATSS_Functional/OperateStation/AutomateCaretaking ==
  Bus Element Out1 : Outport  PortName=ControlCommands

== system CATSS_Functional/OperateStation/CommunicateWithEarth ==

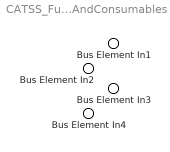
== system CATSS_Functional/OperateStation/ManageAutonomyAndConsumables ==
  Bus Element In1 : Inport  PortName=EnvTelemetry_LifeSupport
  Bus Element In2 : Inport  Port=2  PortName=EnvTelemetry_Habitat
  Bus Element In3 : Inport  Port=3  PortName=ColonyHealthData
  Bus Element In4 : Inport  Port=4  PortName=SafetyState

== system CATSS_Functional/OperateStation/ManageLogisticsAndResupply ==
  Bus Element Out1 : Outport  PortName=Consumables

== system CATSS_Functional/ProvideHabitat/ManageSocialStructure ==

== system CATSS_Functional/ProvideHabitat/ProvideEnrichment ==

== system CATSS_Functional/ProvideHabitat/ProvideTerritoryAndLocomotion ==
  Bus Element In1 : Inport  PortName=ConditionedAtmosphere

== system CATSS_Functional/ProvideHabitat/RegulateSensoryEnvironment ==
  Bus Element In1 : Inport  PortName=ControlCommands
  Bus Element Out1 : Outport  PortName=EnvironmentTelemetry

== system CATSS_Functional/SustainLifeSupport/ControlThermalEnvironment ==

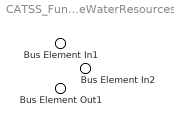
== system CATSS_Functional/SustainLifeSupport/ManageWaterResources ==
  Bus Element In1 : Inport  PortName=WasteStream
  Bus Element In2 : Inport  Port=2  PortName=Consumables
  Bus Element Out1 : Outport  PortName=PotableWater

== system CATSS_Functional/SustainLifeSupport/PurifyCabinAir ==

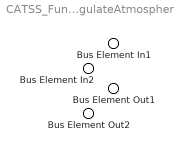
== system CATSS_Functional/SustainLifeSupport/RegulateAtmosphere ==
  Bus Element In1 : Inport  PortName=ControlCommands
  Bus Element In2 : Inport  Port=2  PortName=SafetyState
  Bus Element Out1 : Outport  PortName=ConditionedAtmosphere
  Bus Element Out2 : Outport  Port=2  PortName=EnvironmentTelemetry
